simulink model "ALU_Project"  (R2023b)
settings: Solver=VariableStepAuto  StartTime=0.0  StopTime=1  RelTol=1e-3
values from neighbouring files (symbols this model uses):
  A0 = str2num(get(handles.a0i,'string'))    [AluGui.m]
  A1 = str2num(get(handles.a1i,'string'))    [AluGui.m]
  A2 = str2num(get(handles.a2i,'string'))    [AluGui.m]
  A3 = str2num(get(handles.a3i,'string'))    [AluGui.m]
  B0 = str2num(get(handles.b0i,'string'))    [AluGui.m]
  B1 = str2num(get(handles.b1i,'string'))    [AluGui.m]
  B2 = str2num(get(handles.b2i,'string'))    [AluGui.m]
  B3 = str2num(get(handles.b3i,'string'))    [AluGui.m]
  Cin = str2num(get(handles.cii,'string'))    [AluGui.m]
undefined symbols (not defined in the file or in its folder): S0, S1, S2, S3
(part 1 of 2)
settings Model: Creator=remon  LastModifiedBy=Ibrahim

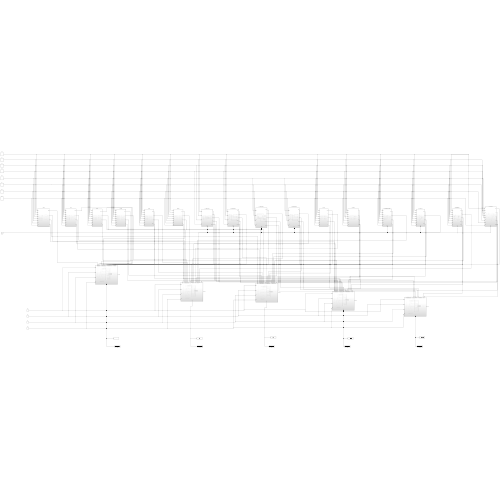
[thumbnail: Simulink's stored preview of the top-level diagram]
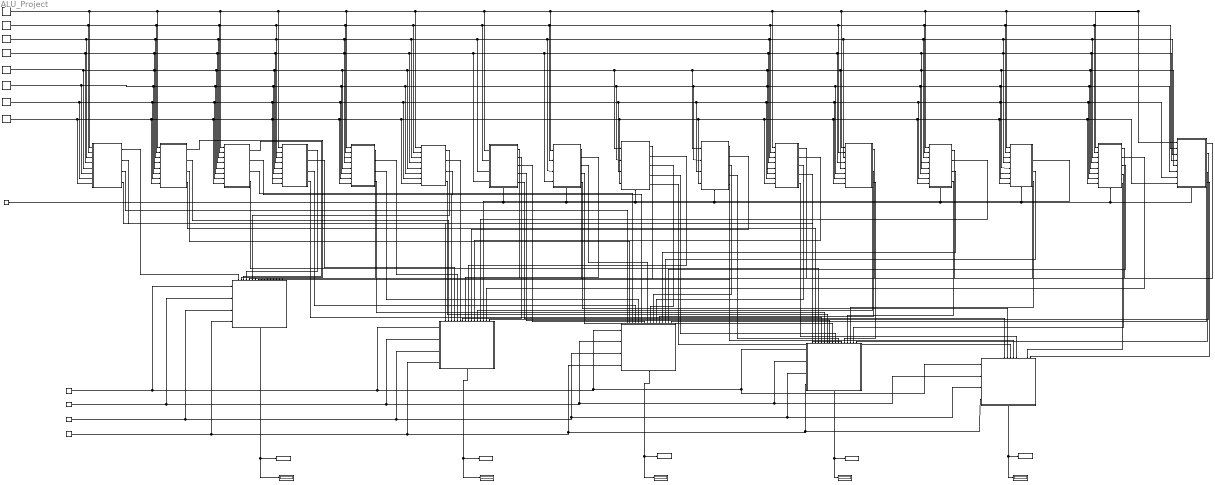
== system ALU_Project ==
  1 AND : Subsystem
  10 -SHIFT RIGHT B : Subsystem
      settings: PortSchema="{\"entries\":[{\"content\":{\"sides\":[{\"content\":{\"connectorIds\":[\"In1\",\"In2\",\"In3\",\"In4\"]},\"type\":\"ConnectorPlacement.EquallySpacedRectSide\",\"uuid\":\"67726d20-445a-49cb-8099-ac09b8ccc5e3\"},{\"content\":{\"connectorIds\":[\"Out1\",\"Out2\",\"Out3\",\"Out4\",\"Out5\"],\"side\":\"RIGHT\"},\"type\":\"ConnectorPlacement.EquallySpacedRectSide\",\"uuid\":\"ee54af08-fb8b-46dc-82ba-e86450b02724\"},{\"content\":{\"side\":\"TOP\"},\"type\":\"ConnectorPlacement.EquallySpacedRectSide\",\"uuid\":\"af06175e-2524-4fad-9974-7a0067daabff\"},{\"content\":{\"connectorIds\":[\"In5\"],\"side\":\"BOTTOM\"},\"type\":\"ConnectorPlacement.EquallySpacedRectSide\",\"uuid\":\"92107ca8-34e5-4b67-bc45-0b30bbde407d\"}]},\"type\":\"ConnectorPlacement.EquallySpacedConnector\",\"uuid\":\"fa9ce2c6-f799-4f73-a92a-f2785f87a999\"}],\"packageUris\":[\"http://schema.mathworks.com/mf0/Connector/R2020b\"],\"version\":\"1.0\"}"
  11 ADD : Subsystem
  12 Subract : Subsystem
  13- SELECTIVE CLEAR : Subsystem
      settings: PortSchema="{\"entries\":[{\"content\":{\"sides\":[{\"content\":{\"connectorIds\":[\"In1\",\"In2\",\"In3\",\"In4\",\"In5\",\"In6\",\"In7\",\"In8\"]},\"type\":\"ConnectorPlacement.EquallySpacedRectSide\",\"uuid\":\"aab1b221-1cb0-4ca9-8866-8bcfb9a4275b\"},{\"content\":{\"connectorIds\":[\"Out1\",\"Out2\",\"Out3\",\"Out4\"],\"side\":\"RIGHT\"},\"type\":\"ConnectorPlacement.EquallySpacedRectSide\",\"uuid\":\"6c2b9ce8-0a07-48e2-b787-5726e3fcf444\"},{\"content\":{\"side\":\"TOP\"},\"type\":\"ConnectorPlacement.EquallySpacedRectSide\",\"uuid\":\"ec29be9f-ac31-4973-a38d-892f27b9a585\"},{\"content\":{\"connectorIds\":[\"In9\"],\"side\":\"BOTTOM\"},\"type\":\"ConnectorPlacement.EquallySpacedRectSide\",\"uuid\":\"88a653d5-a71c-4607-949c-648803d8be5b\"}]},\"type\":\"ConnectorPlacement.EquallySpacedConnector\",\"uuid\":\"295ec8fd-c3b0-41a0-b149-0cfcf8f834a3\"}],\"packageUris\":[\"http://schema.mathworks.com/mf0/Connector/R2020b\"],\"version\":\"1.0\"}"
  14 Compleent : Subsystem
      settings: PortSchema="{\"entries\":[{\"content\":{\"sides\":[{\"content\":{\"connectorIds\":[\"In1\",\"In2\",\"In3\",\"In4\",\"In5\",\"In6\",\"In7\",\"In8\"]},\"type\":\"ConnectorPlacement.EquallySpacedRectSide\",\"uuid\":\"aab1b221-1cb0-4ca9-8866-8bcfb9a4275b\"},{\"content\":{\"connectorIds\":[\"Out1\",\"Out2\",\"Out3\",\"Out4\"],\"side\":\"RIGHT\"},\"type\":\"ConnectorPlacement.EquallySpacedRectSide\",\"uuid\":\"6c2b9ce8-0a07-48e2-b787-5726e3fcf444\"},{\"content\":{\"side\":\"TOP\"},\"type\":\"ConnectorPlacement.EquallySpacedRectSide\",\"uuid\":\"ec29be9f-ac31-4973-a38d-892f27b9a585\"},{\"content\":{\"connectorIds\":[\"In9\"],\"side\":\"BOTTOM\"},\"type\":\"ConnectorPlacement.EquallySpacedRectSide\",\"uuid\":\"df039325-7ad8-41a5-924c-b29ed495d143\"}]},\"type\":\"ConnectorPlacement.EquallySpacedConnector\",\"uuid\":\"295ec8fd-c3b0-41a0-b149-0cfcf8f834a3\"}],\"packageUris\":[\"http://schema.mathworks.com/mf0/Connector/R2020b\"],\"version\":\"1.0\"}"
  15-DECREMENT : Subsystem
      settings: PortSchema="{\"entries\":[{\"content\":{\"sides\":[{\"content\":{\"connectorIds\":[\"In1\",\"In2\",\"In3\",\"In4\",\"In5\",\"In6\",\"In7\",\"In8\"]},\"type\":\"ConnectorPlacement.EquallySpacedRectSide\",\"uuid\":\"869fb0d4-d1f3-44bd-a919-19db4d026c4c\"},{\"content\":{\"connectorIds\":[\"Out1\",\"Out2\",\"Out3\",\"Out4\",\"Out5\"],\"side\":\"RIGHT\"},\"type\":\"ConnectorPlacement.EquallySpacedRectSide\",\"uuid\":\"d1e23600-62c0-4a53-bf3f-03977fd433f6\"},{\"content\":{\"side\":\"TOP\"},\"type\":\"ConnectorPlacement.EquallySpacedRectSide\",\"uuid\":\"a43d6e83-8d01-47cf-bcfd-6ee8cba25de0\"},{\"content\":{\"connectorIds\":[\"In9\"],\"side\":\"BOTTOM\"},\"type\":\"ConnectorPlacement.EquallySpacedRectSide\",\"uuid\":\"b69fe367-260d-455e-bab1-d94656d66442\"}]},\"type\":\"ConnectorPlacement.EquallySpacedConnector\",\"uuid\":\"60700526-3682-4bd8-a800-7fae9f1c6513\"}],\"packageUris\":[\"http://schema.mathworks.com/mf0/Connector/R2020b\"],\"version\":\"1.0\"}"
  16 -Increment : Subsystem
      settings: PortSchema="{\"entries\":[{\"content\":{\"sides\":[{\"content\":{\"connectorIds\":[\"In1\",\"In2\",\"In3\",\"In4\",\"In5\",\"In6\",\"In7\",\"In8\"]},\"type\":\"ConnectorPlacement.EquallySpacedRectSide\",\"uuid\":\"3ea3efc1-2c41-45a7-8c9d-434968181f92\"},{\"content\":{\"connectorIds\":[\"Out1\",\"Out2\",\"Out3\",\"Out4\",\"Out5\"],\"side\":\"RIGHT\"},\"type\":\"ConnectorPlacement.EquallySpacedRectSide\",\"uuid\":\"65b61c40-0cda-4050-95e7-78f124d34506\"},{\"content\":{\"side\":\"TOP\"},\"type\":\"ConnectorPlacement.EquallySpacedRectSide\",\"uuid\":\"defff18e-4aec-4535-bbe1-adefcaebceb1\"},{\"content\":{\"connectorIds\":[\"In9\"],\"side\":\"BOTTOM\"},\"type\":\"ConnectorPlacement.EquallySpacedRectSide\",\"uuid\":\"2835e909-4c73-48e4-9b82-396162bc7647\"}]},\"type\":\"ConnectorPlacement.EquallySpacedConnector\",\"uuid\":\"844f857b-b7f5-4d2c-b420-0fa89070e8b7\"}],\"packageUris\":[\"http://schema.mathworks.com/mf0/Connector/R2020b\"],\"version\":\"1.0\"}"
  2 OR : Subsystem
  3 NOR : Subsystem
  4 NAND : Subsystem
  5 XOR : Subsystem
  6 XNOR : Subsystem
  7 - A SHFIT LEFT : Subsystem
      settings: PortSchema="{\"entries\":[{\"content\":{\"sides\":[{\"content\":{\"connectorIds\":[\"In1\",\"In2\",\"In3\",\"In4\"]},\"type\":\"ConnectorPlacement.EquallySpacedRectSide\",\"uuid\":\"67726d20-445a-49cb-8099-ac09b8ccc5e3\"},{\"content\":{\"connectorIds\":[\"Out1\",\"Out2\",\"Out3\",\"Out4\",\"Out5\"],\"side\":\"RIGHT\"},\"type\":\"ConnectorPlacement.EquallySpacedRectSide\",\"uuid\":\"ee54af08-fb8b-46dc-82ba-e86450b02724\"},{\"content\":{\"side\":\"TOP\"},\"type\":\"ConnectorPlacement.EquallySpacedRectSide\",\"uuid\":\"af06175e-2524-4fad-9974-7a0067daabff\"},{\"content\":{\"connectorIds\":[\"In5\"],\"side\":\"BOTTOM\"},\"type\":\"ConnectorPlacement.EquallySpacedRectSide\",\"uuid\":\"f9a8dd3b-7a22-45bd-9502-add1c2d213e4\"}]},\"type\":\"ConnectorPlacement.EquallySpacedConnector\",\"uuid\":\"fa9ce2c6-f799-4f73-a92a-f2785f87a999\"}],\"packageUris\":[\"http://schema.mathworks.com/mf0/Connector/R2020b\"],\"version\":\"1.0\"}"
  8 - SHIFT RIGHT A : Subsystem
      settings: PortSchema="{\"entries\":[{\"content\":{\"sides\":[{\"content\":{\"connectorIds\":[\"In1\",\"In2\",\"In3\",\"In4\"]},\"type\":\"ConnectorPlacement.EquallySpacedRectSide\",\"uuid\":\"67726d20-445a-49cb-8099-ac09b8ccc5e3\"},{\"content\":{\"connectorIds\":[\"Out1\",\"Out2\",\"Out3\",\"Out4\",\"Out5\"],\"side\":\"RIGHT\"},\"type\":\"ConnectorPlacement.EquallySpacedRectSide\",\"uuid\":\"ee54af08-fb8b-46dc-82ba-e86450b02724\"},{\"content\":{\"side\":\"TOP\"},\"type\":\"ConnectorPlacement.EquallySpacedRectSide\",\"uuid\":\"af06175e-2524-4fad-9974-7a0067daabff\"},{\"content\":{\"connectorIds\":[\"In5\"],\"side\":\"BOTTOM\"},\"type\":\"ConnectorPlacement.EquallySpacedRectSide\",\"uuid\":\"c41446c6-b653-4be8-be63-43ab09cffb18\"}]},\"type\":\"ConnectorPlacement.EquallySpacedConnector\",\"uuid\":\"fa9ce2c6-f799-4f73-a92a-f2785f87a999\"}],\"packageUris\":[\"http://schema.mathworks.com/mf0/Connector/R2020b\"],\"version\":\"1.0\"}"
  "9 - B SHIFT LEFT " : Subsystem
      settings: PortSchema="{\"entries\":[{\"content\":{\"sides\":[{\"content\":{\"connectorIds\":[\"In1\",\"In2\",\"In3\",\"In4\"]},\"type\":\"ConnectorPlacement.EquallySpacedRectSide\",\"uuid\":\"67726d20-445a-49cb-8099-ac09b8ccc5e3\"},{\"content\":{\"connectorIds\":[\"Out1\",\"Out2\",\"Out3\",\"Out4\",\"Out5\"],\"side\":\"RIGHT\"},\"type\":\"ConnectorPlacement.EquallySpacedRectSide\",\"uuid\":\"ee54af08-fb8b-46dc-82ba-e86450b02724\"},{\"content\":{\"side\":\"TOP\"},\"type\":\"ConnectorPlacement.EquallySpacedRectSide\",\"uuid\":\"af06175e-2524-4fad-9974-7a0067daabff\"},{\"content\":{\"connectorIds\":[\"In5\"],\"side\":\"BOTTOM\"},\"type\":\"ConnectorPlacement.EquallySpacedRectSide\",\"uuid\":\"689fe6fd-fd8e-4c12-8b2b-d8e14b2aa840\"}]},\"type\":\"ConnectorPlacement.EquallySpacedConnector\",\"uuid\":\"fa9ce2c6-f799-4f73-a92a-f2785f87a999\"}],\"packageUris\":[\"http://schema.mathworks.com/mf0/Connector/R2020b\"],\"version\":\"1.0\"}"
  A0 : Constant  Value=A0
  A1 : Constant  Value=A1
  A2 : Constant  Value=A2
  A3 : Constant  Value=A3
  B0 : Constant  Value=B0
  B1 : Constant  Value=B1
  B2 : Constant  Value=B2
  B3 : Constant  Value=B3
  CIn : Constant  Value=Cin
  Cout : Display
  S0 : Constant  Value=S0
  S1 : Constant  Value=S1
  S2 : Constant  Value=S2
  S3 : Constant  Value=S3
  To Workspace : ToWorkspace  VariableName=Z2  SampleTime=-1
  To Workspace1 : ToWorkspace  VariableName=Z3  SampleTime=-1
  To Workspace2 : ToWorkspace  VariableName=Cout  SampleTime=-1
  To Workspace3 : ToWorkspace  VariableName=Z1  SampleTime=-1
  To Workspace4 : ToWorkspace  VariableName=Z0  SampleTime=-1
  Z0 : Display
  "Z1 " : Display
  Z2 : Display
  Z3 : Display
  bit 1 out : Subsystem
      settings: PortSchema="{\"entries\":[{\"content\":{\"sides\":[{\"content\":{\"connectorIds\":[\"In1\",\"In2\",\"In3\",\"In4\",\"In5\",\"In6\",\"In7\",\"In8\",\"In9\",\"In10\",\"In11\",\"In12\",\"In13\",\"In14\",\"In15\",\"In16\"]},\"type\":\"ConnectorPlacement.EquallySpacedRectSide\",\"uuid\":\"53e370e5-cc10-417f-a084-3353bc2b3524\"},{\"content\":{\"connectorIds\":[\"Out1\"],\"side\":\"RIGHT\"},\"type\":\"ConnectorPlacement.EquallySpacedRectSide\",\"uuid\":\"f2d13301-e5be-4569-a8f2-18325db28854\"},{\"content\":{\"connectorIds\":[\"In17\",\"In18\",\"In19\",\"In20\"],\"side\":\"TOP\"},\"type\":\"ConnectorPlacement.EquallySpacedRectSide\",\"uuid\":\"c3b20576-f5d0-4622-8370-994c765f463a\"}]},\"type\":\"ConnectorPlacement.EquallySpacedConnector\",\"uuid\":\"4e1c3be4-ed9a-414f-b6f4-4528b145bb15\"}],\"packageUris\":[\"http://schema.mathworks.com/mf0/Connector/R2020b\"],\"version\":\"1.0\"}"
  bit 2 out : Subsystem
      settings: PortSchema="{\"entries\":[{\"content\":{\"sides\":[{\"content\":{\"connectorIds\":[\"In1\",\"In2\",\"In3\",\"In4\",\"In5\",\"In6\",\"In7\",\"In8\",\"In9\",\"In10\",\"In11\",\"In12\",\"In13\",\"In14\",\"In15\",\"In16\"]},\"type\":\"ConnectorPlacement.EquallySpacedRectSide\",\"uuid\":\"53e370e5-cc10-417f-a084-3353bc2b3524\"},{\"content\":{\"connectorIds\":[\"Out1\"],\"side\":\"RIGHT\"},\"type\":\"ConnectorPlacement.EquallySpacedRectSide\",\"uuid\":\"f2d13301-e5be-4569-a8f2-18325db28854\"},{\"content\":{\"connectorIds\":[\"In17\",\"In18\",\"In19\",\"In20\"],\"side\":\"TOP\"},\"type\":\"ConnectorPlacement.EquallySpacedRectSide\",\"uuid\":\"c3b20576-f5d0-4622-8370-994c765f463a\"}]},\"type\":\"ConnectorPlacement.EquallySpacedConnector\",\"uuid\":\"4e1c3be4-ed9a-414f-b6f4-4528b145bb15\"}],\"packageUris\":[\"http://schema.mathworks.com/mf0/Connector/R2020b\"],\"version\":\"1.0\"}"
  bit 3 out : Subsystem
      settings: PortSchema="{\"entries\":[{\"content\":{\"sides\":[{\"content\":{\"connectorIds\":[\"In1\",\"In2\",\"In3\",\"In4\",\"In5\",\"In6\",\"In7\",\"In8\",\"In9\",\"In10\",\"In11\",\"In12\",\"In13\",\"In14\",\"In15\",\"In16\"]},\"type\":\"ConnectorPlacement.EquallySpacedRectSide\",\"uuid\":\"53e370e5-cc10-417f-a084-3353bc2b3524\"},{\"content\":{\"connectorIds\":[\"Out1\"],\"side\":\"RIGHT\"},\"type\":\"ConnectorPlacement.EquallySpacedRectSide\",\"uuid\":\"f2d13301-e5be-4569-a8f2-18325db28854\"},{\"content\":{\"connectorIds\":[\"In17\",\"In18\",\"In19\",\"In20\"],\"side\":\"TOP\"},\"type\":\"ConnectorPlacement.EquallySpacedRectSide\",\"uuid\":\"c3b20576-f5d0-4622-8370-994c765f463a\"}]},\"type\":\"ConnectorPlacement.EquallySpacedConnector\",\"uuid\":\"4e1c3be4-ed9a-414f-b6f4-4528b145bb15\"}],\"packageUris\":[\"http://schema.mathworks.com/mf0/Connector/R2020b\"],\"version\":\"1.0\"}"
  bit 4 out : Subsystem
      settings: PortSchema="{\"entries\":[{\"content\":{\"sides\":[{\"content\":{\"connectorIds\":[\"In1\",\"In2\",\"In3\",\"In4\",\"In5\",\"In6\",\"In7\",\"In8\",\"In9\",\"In10\",\"In11\",\"In12\",\"In13\",\"In14\",\"In15\",\"In16\"]},\"type\":\"ConnectorPlacement.EquallySpacedRectSide\",\"uuid\":\"53e370e5-cc10-417f-a084-3353bc2b3524\"},{\"content\":{\"connectorIds\":[\"Out1\"],\"side\":\"RIGHT\"},\"type\":\"ConnectorPlacement.EquallySpacedRectSide\",\"uuid\":\"f2d13301-e5be-4569-a8f2-18325db28854\"},{\"content\":{\"connectorIds\":[\"In17\",\"In18\",\"In19\",\"In20\"],\"side\":\"TOP\"},\"type\":\"ConnectorPlacement.EquallySpacedRectSide\",\"uuid\":\"c3b20576-f5d0-4622-8370-994c765f463a\"}]},\"type\":\"ConnectorPlacement.EquallySpacedConnector\",\"uuid\":\"4e1c3be4-ed9a-414f-b6f4-4528b145bb15\"}],\"packageUris\":[\"http://schema.mathworks.com/mf0/Connector/R2020b\"],\"version\":\"1.0\"}"
  bit Cout : Subsystem
      settings: PortSchema="{\"entries\":[{\"content\":{\"sides\":[{\"content\":{\"connectorIds\":[\"In1\",\"In2\",\"In3\",\"In4\",\"In5\",\"In6\",\"In7\",\"In8\",\"In9\",\"In10\",\"In11\",\"In12\",\"In13\",\"In14\",\"In15\",\"In16\"]},\"type\":\"ConnectorPlacement.EquallySpacedRectSide\",\"uuid\":\"53e370e5-cc10-417f-a084-3353bc2b3524\"},{\"content\":{\"connectorIds\":[\"Out1\"],\"side\":\"RIGHT\"},\"type\":\"ConnectorPlacement.EquallySpacedRectSide\",\"uuid\":\"f2d13301-e5be-4569-a8f2-18325db28854\"},{\"content\":{\"connectorIds\":[\"In17\",\"In18\",\"In19\",\"In20\"],\"side\":\"TOP\"},\"type\":\"ConnectorPlacement.EquallySpacedRectSide\",\"uuid\":\"c3b20576-f5d0-4622-8370-994c765f463a\"}]},\"type\":\"ConnectorPlacement.EquallySpacedConnector\",\"uuid\":\"4e1c3be4-ed9a-414f-b6f4-4528b145bb15\"}],\"packageUris\":[\"http://schema.mathworks.com/mf0/Connector/R2020b\"],\"version\":\"1.0\"}"
  wires:
  B1/1 -> 1 AND/6(B1), 2 OR/6(B1), 4 NAND/6(B1), 5 XOR/6(B1), 6 XNOR/6(B1), "9 - B SHIFT LEFT "/2(B1), 10 -SHIFT RIGHT B/2(B1), 11 ADD/6(B1), 12 Subract/6(B1), 13- SELECTIVE CLEAR/6(B1), 14 Compleent/6(B1), 15-DECREMENT/6(B1), 16 -Increment/6(B1), 3 NOR/6(B1)
  A3/1 -> 1 AND/4(A3), 2 OR/4(A3), 4 NAND/4(A3), 5 XOR/4(A3), 6 XNOR/4(A3), 7 - A SHFIT LEFT/4(A3), 8 - SHIFT RIGHT A/4(A3), 11 ADD/4(A3), 12 Subract/4(A3), 13- SELECTIVE CLEAR/4(A3), 14 Compleent/4(A3), 15-DECREMENT/4(A3), 16 -Increment/4(A3), 3 NOR/4(A3)
  B3/1 -> 1 AND/8(B3), 2 OR/8(B3), 4 NAND/8(B3), 6 XNOR/8(B3), "9 - B SHIFT LEFT "/4(B3), 10 -SHIFT RIGHT B/4(B3), 11 ADD/8(B3), 12 Subract/8(B3), 13- SELECTIVE CLEAR/8(B3), 14 Compleent/8(B3), 15-DECREMENT/8(B3), 16 -Increment/8(B3), 5 XOR/8(B3), 3 NOR/8(B3)
  B2/1 -> 1 AND/7(B2), 2 OR/7(B2), 4 NAND/7(B2), 5 XOR/7(B2), 6 XNOR/7(B2), "9 - B SHIFT LEFT "/3(B2), 10 -SHIFT RIGHT B/3(B2), 11 ADD/7(B2), 12 Subract/7(B2), 13- SELECTIVE CLEAR/7(B2), 14 Compleent/7(B2), 15-DECREMENT/7(B2), 16 -Increment/7(B2), 3 NOR/7(B2)
  A1/1 -> 1 AND/2(A1), 2 OR/2(A1), 4 NAND/2(A1), 6 XNOR/2(A1), 7 - A SHFIT LEFT/2(A1), 8 - SHIFT RIGHT A/2(A1), 13- SELECTIVE CLEAR/2(A1), 16 -Increment/2(A1), 15-DECREMENT/2(A1), 14 Compleent/2(A1), 12 Subract/2(A1), 11 ADD/2(A1), 5 XOR/2(A1), 3 NOR/2(A1)
  B0/1 -> 1 AND/5(B0), 2 OR/5(B0), 4 NAND/5(B0), 5 XOR/5(B0), 6 XNOR/5(B0), "9 - B SHIFT LEFT "/1(B0), 10 -SHIFT RIGHT B/1(B0), 11 ADD/5(B0), 14 Compleent/5(B0), 15-DECREMENT/5(B0), 16 -Increment/5(B0), 13- SELECTIVE CLEAR/5(B0), 12 Subract/5(B0), 3 NOR/5(B0)
  A2/1 -> 1 AND/3(A2), 2 OR/3(A2), 4 NAND/3(A2), 5 XOR/3(A2), 6 XNOR/3(A2), 7 - A SHFIT LEFT/3(A2), 8 - SHIFT RIGHT A/3(A2), 11 ADD/3(A2), 12 Subract/3(A2), 14 Compleent/3(A2), 15-DECREMENT/3(A2), 16 -Increment/3(A2), 13- SELECTIVE CLEAR/3(A2), 3 NOR/3(A2)
  A0/1 -> 1 AND/1(A0), 2 OR/1(A0), 4 NAND/1(A0), 5 XOR/1(A0), 6 XNOR/1(A0), 7 - A SHFIT LEFT/1(A0), 8 - SHIFT RIGHT A/1(A0), 11 ADD/1(A0), 12 Subract/1(A0), 13- SELECTIVE CLEAR/1(A0), 14 Compleent/1(A0), 16 -Increment/1(A0), 15-DECREMENT/1(A0), 3 NOR/1(A0)
  CIn/1 -> 8 - SHIFT RIGHT A/5(CIN), 13- SELECTIVE CLEAR/9(CIN), 16 -Increment/9(Cin), 15-DECREMENT/9(Cin), 14 Compleent/9(Cin), 10 -SHIFT RIGHT B/5(CIN), "9 - B SHIFT LEFT "/5(CIN), 7 - A SHFIT LEFT/5(CIN)
  1 AND/1(0000) -> bit 1 out/1(0000)
  2 OR/1(0001) -> bit 1 out/2(0001)
  3 NOR/1(0010) -> bit 1 out/3(0010)
  4 NAND/1(0011) -> bit 1 out/4(0011)
  5 XOR/1(0100) -> bit 1 out/5(0100)
  6 XNOR/1(0101) -> bit 1 out/6(0101)
  7 - A SHFIT LEFT/1(1) -> bit 1 out/7(0110)
  8 - SHIFT RIGHT A/1(0111) -> bit 1 out/8(0111)
  "9 - B SHIFT LEFT "/1(1000) -> bit 1 out/9(1000)
  10 -SHIFT RIGHT B/1(1001) -> bit 1 out/10(1001)
  11 ADD/1(1010) -> bit 1 out/11(1010)
  12 Subract/1(1) -> bit 1 out/12(1011)
  13- SELECTIVE CLEAR/1(1100) -> bit 1 out/13(1100)
  14 Compleent/1(1101) -> bit 1 out/14(1101)
  15-DECREMENT/1(1110) -> bit 1 out/15(1110)
  16 -Increment/1(1111) -> bit 1 out/16(1111)
  1 AND/2(Out2) -> bit 2 out/1(0000)
  2 OR/2(Out2) -> bit 2 out/2(0001)
  3 NOR/2(Out2) -> bit 2 out/3(0010)
  4 NAND/2(Out2) -> bit 2 out/4(0011)
  5 XOR/2(Out2) -> bit 2 out/5(0100)
  6 XNOR/2(Out2) -> bit 2 out/6(0101)
  7 - A SHFIT LEFT/2(2) -> bit 2 out/7(0110)
  8 - SHIFT RIGHT A/2(Out2) -> bit 2 out/8(0111)
  "9 - B SHIFT LEFT "/2(Out2) -> bit 2 out/9(1000)
  10 -SHIFT RIGHT B/2(Out2) -> bit 2 out/10(1001)
  11 ADD/2(Out2) -> bit 2 out/11(1010)
  12 Subract/2(Out2) -> bit 2 out/12(1011)
  13- SELECTIVE CLEAR/2(Out2) -> bit 2 out/13(1100)
  14 Compleent/2(Out2) -> bit 2 out/14(1101)
  15-DECREMENT/2(Out2) -> bit 2 out/15(1110)
  16 -Increment/2(Out2) -> bit 2 out/16(1111)
  1 AND/3(Out3) -> bit 3 out/1(0000)
  2 OR/3(Out3) -> bit 3 out/2(0001)
  3 NOR/3(Out3) -> bit 3 out/3(0010)
  4 NAND/3(Out3) -> bit 3 out/4(0011)
  5 XOR/3(Out3) -> bit 3 out/5(0100)
  6 XNOR/3(Out3) -> bit 3 out/6(0101)
  7 - A SHFIT LEFT/3(3) -> bit 3 out/7(0110)
  8 - SHIFT RIGHT A/3(Out3) -> bit 3 out/8(0111)
  "9 - B SHIFT LEFT "/3(Out3) -> bit 3 out/9(1000)
  10 -SHIFT RIGHT B/3(Out3) -> bit 3 out/10(1001)
  11 ADD/3(Out3) -> bit 3 out/11(1010)
  12 Subract/3(Out3) -> bit 3 out/12(1011)
  13- SELECTIVE CLEAR/3(Out3) -> bit 3 out/13(1100)
  14 Compleent/3(Out3) -> bit 3 out/14(1101)
  15-DECREMENT/3(Out3) -> bit 3 out/15(1110)
  16 -Increment/3(Out3) -> bit 3 out/16(1111)
  1 AND/4(Out4) -> bit 4 out/1(0000)
  2 OR/4(Out4) -> bit 4 out/2(0001)
  3 NOR/4(Out4) -> bit 4 out/3(0010)
  4 NAND/4(Out4) -> bit 4 out/4(0011)
  5 XOR/4(0101) -> bit 4 out/5(0100)
  6 XNOR/4(Out4) -> bit 4 out/6(0101)
  7 - A SHFIT LEFT/4(" 4") -> bit 4 out/7(0110)
  8 - SHIFT RIGHT A/4(Out 4) -> bit 4 out/8(0111)
  "9 - B SHIFT LEFT "/4(Out 4) -> bit 4 out/9(1000)
  10 -SHIFT RIGHT B/4(Out 4) -> bit 4 out/10(1001)
  11 ADD/4(Out4) -> bit 4 out/11(1010)
  12 Subract/4(Out4) -> bit 4 out/12(1011)
  13- SELECTIVE CLEAR/4(Out4) -> bit 4 out/13(1100)
  14 Compleent/4(1100) -> bit 4 out/14(1101)
  15-DECREMENT/4(1101) -> bit 4 out/15(1110)
  16 -Increment/4(Out4) -> bit 4 out/16(1111)
  7 - A SHFIT LEFT/5(COUT) -> bit Cout/7(0110)
  8 - SHIFT RIGHT A/5(COUT) -> bit Cout/8(0111)
  "9 - B SHIFT LEFT "/5(COUT) -> bit Cout/9(1000)
  10 -SHIFT RIGHT B/5(COUT) -> bit Cout/10(1001)
  15-DECREMENT/5(Cout) -> bit Cout/15(1110)
  16 -Increment/5(Cout) -> bit Cout/16(1111)
  bit Cout/1(Out) -> Cout/1, To Workspace2/1
  bit 4 out/1(Out) -> To Workspace1/1, Z3/1
  bit 3 out/1(Out) -> To Workspace/1, Z2/1
  bit 2 out/1(Out) -> To Workspace3/1, "Z1 "/1
  bit 1 out/1(Out) -> To Workspace4/1, Z0/1
  S3/1 -> bit 1 out/17(S3), bit 2 out/17(S3), bit Cout/17(S3), bit 4 out/17(S3), bit 3 out/17(S3)
  S2/1 -> bit 1 out/18(S2), bit 2 out/18(S2), bit Cout/18(S2), bit 4 out/18(S2), bit 3 out/18(S2)
  S1/1 -> bit 1 out/19(S1), bit 2 out/19(S1), bit 3 out/19(S1), bit Cout/19(S1), bit 4 out/19(S1)
  S0/1 -> bit 2 out/20(S0), bit 3 out/20(S0), bit 4 out/20(S0), bit Cout/20(S0), bit 1 out/20(S0)
  11 ADD/5(Out5) -> bit Cout/11(1010)

== system ALU_Project/1 AND ==
  A0 : Inport
  A1 : Inport  Port=2
  A2 : Inport  Port=3
  A3 : Inport  Port=4
  B0 : Inport  Port=5
  B1 : Inport  Port=6
  B2 : Inport  Port=7
  B3 : Inport  Port=8
   {,1..3} (4 alike) : Logic  AllPortsSameDT=off  OutDataTypeStr=boolean
  display{,1..3} (4 alike) : Display
  0000 : Outport
  Out2 : Outport  Port=2
  Out3 : Outport  Port=3
  Out4 : Outport  Port=4
  wires:
  A0/1 -> " "/1
  B0/1 -> " "/2
  A1/1 -> " 1"/1
  B1/1 -> " 1"/2
  A2/1 -> " 2"/1
  B2/1 -> " 2"/2
  A3/1 -> " 3"/1
  B3/1 -> " 3"/2
  " 1"/1 -> Out2/1, display1/1
  " "/1 -> 0000/1, display/1
  " 3"/1 -> Out4/1, display3/1
  " 2"/1 -> Out3/1, display2/1

== system ALU_Project/10 -SHIFT RIGHT B ==
  B0 : Inport
  B1 : Inport  Port=2
  B2 : Inport  Port=3
  B3 : Inport  Port=4
  CIN : Inport  Port=5
  1001 : Outport
  Out2 : Outport  Port=2
  Out3 : Outport  Port=3
  Out 4 : Outport  Port=4
  COUT : Outport  Port=5
  wires:
  B3/1 -> Out3/1
  CIN/1 -> Out 4/1
  B2/1 -> Out2/1
  B1/1 -> 1001/1
  B0/1 -> COUT/1

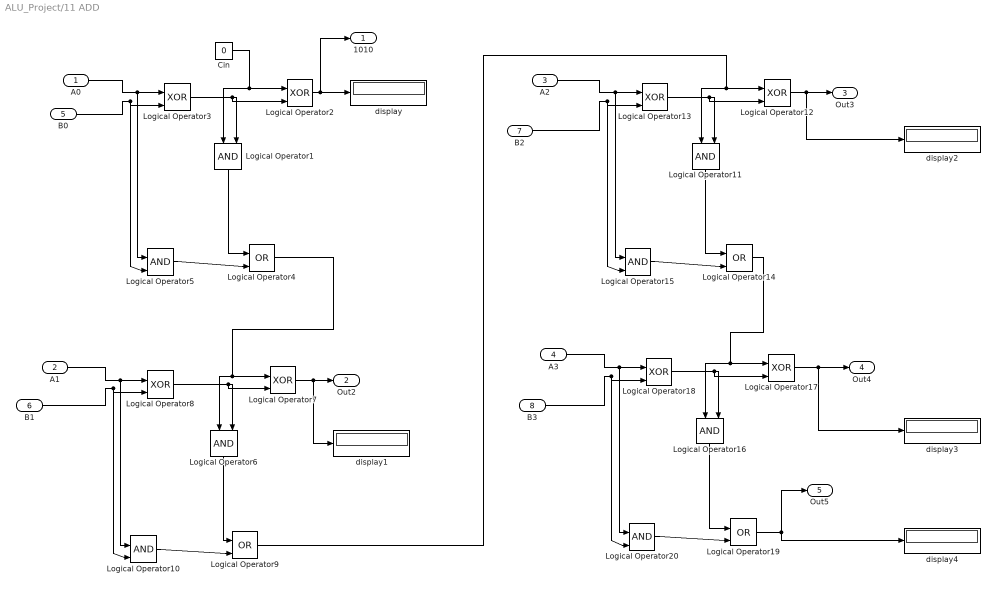
== system ALU_Project/11 ADD ==
  A0 : Inport
  A1 : Inport  Port=2
  A2 : Inport  Port=3
  A3 : Inport  Port=4
  B0 : Inport  Port=5
  B1 : Inport  Port=6
  B2 : Inport  Port=7
  B3 : Inport  Port=8
  Cin : Constant  Value=0
  Logical Operator{1,5..6,10..11,15..16,20} (8 alike) : Logic  IconShape=distinctive  AllPortsSameDT=off  OutDataTypeStr=boolean
  Logical Operator{2..3,7..8,12..13,17..18} (8 alike) : Logic  Operator=XOR  IconShape=distinctive  AllPortsSameDT=off  OutDataTypeStr=boolean
  Logical Operator{4,9,14,19} (4 alike) : Logic  Operator=OR  IconShape=distinctive  AllPortsSameDT=off  OutDataTypeStr=boolean
  display{,1..4} (5 alike) : Display
  1010 : Outport
  Out2 : Outport  Port=2
  Out3 : Outport  Port=3
  Out4 : Outport  Port=4
  Out5 : Outport  Port=5
  wires:
  Logical Operator3/1 -> Logical Operator2/2, Logical Operator1/2
  Logical Operator1/1 -> Logical Operator4/1
  Logical Operator5/1 -> Logical Operator4/2
  B0/1 -> Logical Operator5/2, Logical Operator3/2
  Cin/1 -> Logical Operator1/1, Logical Operator2/1
  Logical Operator2/1 -> display/1, 1010/1
  A0/1 -> Logical Operator5/1, Logical Operator3/1
  Logical Operator8/1 -> Logical Operator7/2, Logical Operator6/2
  Logical Operator6/1 -> Logical Operator9/1
  Logical Operator10/1 -> Logical Operator9/2
  B1/1 -> Logical Operator10/2, Logical Operator8/2
  Logical Operator4/1 -> Logical Operator6/1, Logical Operator7/1
  Logical Operator7/1 -> display1/1, Out2/1
  A1/1 -> Logical Operator10/1, Logical Operator8/1
  Logical Operator13/1 -> Logical Operator12/2, Logical Operator11/2
  Logical Operator11/1 -> Logical Operator14/1
  Logical Operator15/1 -> Logical Operator14/2
  B2/1 -> Logical Operator15/2, Logical Operator13/2
  Logical Operator9/1 -> Logical Operator11/1, Logical Operator12/1
  A2/1 -> Logical Operator15/1, Logical Operator13/1
  Logical Operator18/1 -> Logical Operator17/2, Logical Operator16/2
  Logical Operator16/1 -> Logical Operator19/1
  Logical Operator20/1 -> Logical Operator19/2
  B3/1 -> Logical Operator20/2, Logical Operator18/2
  Logical Operator14/1 -> Logical Operator16/1, Logical Operator17/1
  A3/1 -> Logical Operator20/1, Logical Operator18/1
  Logical Operator12/1 -> display2/1, Out3/1
  Logical Operator17/1 -> display3/1, Out4/1
  Logical Operator19/1 -> Out5/1, display4/1

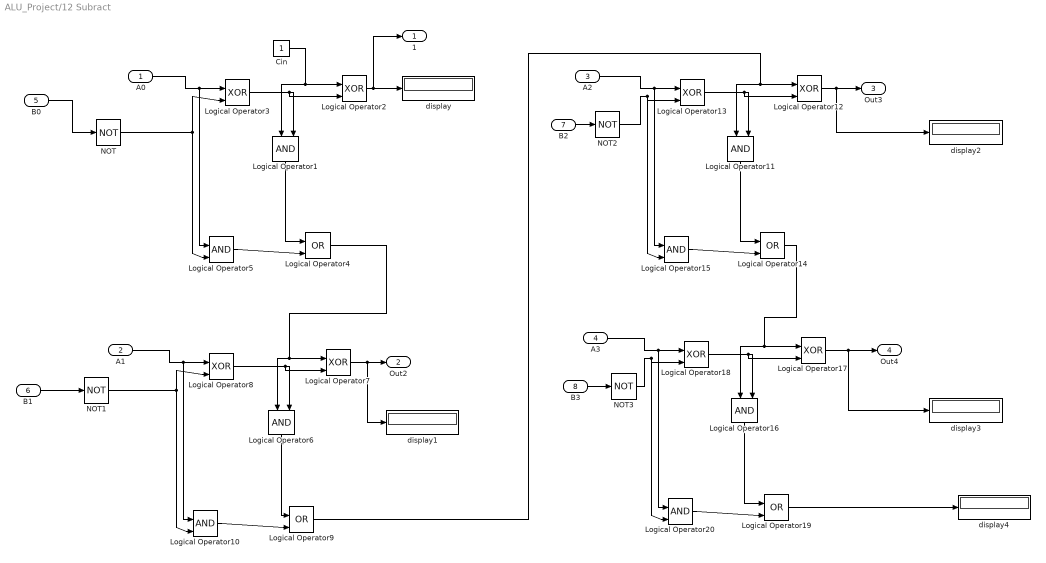
== system ALU_Project/12 Subract ==
  A0 : Inport
  A1 : Inport  Port=2
  A2 : Inport  Port=3
  A3 : Inport  Port=4
  B0 : Inport  Port=5
  B1 : Inport  Port=6
  B2 : Inport  Port=7
  B3 : Inport  Port=8
  Cin : Constant
  Logical Operator{1,5..6,10..11,15..16,20} (8 alike) : Logic  IconShape=distinctive  AllPortsSameDT=off  OutDataTypeStr=boolean
  Logical Operator{2..3,7..8,12..13,17..18} (8 alike) : Logic  Operator=XOR  IconShape=distinctive  AllPortsSameDT=off  OutDataTypeStr=boolean
  Logical Operator{4,9,14,19} (4 alike) : Logic  Operator=OR  IconShape=distinctive  AllPortsSameDT=off  OutDataTypeStr=boolean
  NOT{,1..3} (4 alike) : Logic  Operator=NOT  IconShape=distinctive  AllPortsSameDT=off  OutDataTypeStr=boolean
  display{,1..4} (5 alike) : Display
  1 : Outport
  Out2 : Outport  Port=2
  Out3 : Outport  Port=3
  Out4 : Outport  Port=4
  wires:
  Logical Operator9/1 -> Logical Operator11/1, Logical Operator12/1
  A3/1 -> Logical Operator20/1, Logical Operator18/1
  Logical Operator7/1 -> display1/1, Out2/1
  A0/1 -> Logical Operator5/1, Logical Operator3/1
  B2/1 -> NOT2/1
  Logical Operator14/1 -> Logical Operator16/1, Logical Operator17/1
  B3/1 -> NOT3/1
  A1/1 -> Logical Operator10/1, Logical Operator8/1
  Logical Operator19/1 -> display4/1
  Logical Operator4/1 -> Logical Operator6/1, Logical Operator7/1
  Logical Operator12/1 -> display2/1, Out3/1
  Logical Operator13/1 -> Logical Operator12/2, Logical Operator11/2
  Logical Operator16/1 -> Logical Operator19/1
  Logical Operator18/1 -> Logical Operator17/2, Logical Operator16/2
  A2/1 -> Logical Operator15/1, Logical Operator13/1
  Logical Operator8/1 -> Logical Operator7/2, Logical Operator6/2
  B1/1 -> NOT1/1
  Logical Operator15/1 -> Logical Operator14/2
  Logical Operator11/1 -> Logical Operator14/1
  Logical Operator5/1 -> Logical Operator4/2
  Logical Operator3/1 -> Logical Operator2/2, Logical Operator1/2
  Cin/1 -> Logical Operator1/1, Logical Operator2/1
  Logical Operator10/1 -> Logical Operator9/2
  Logical Operator17/1 -> display3/1, Out4/1
  Logical Operator20/1 -> Logical Operator19/2
  Logical Operator6/1 -> Logical Operator9/1
  B0/1 -> NOT/1
  Logical Operator1/1 -> Logical Operator4/1
  Logical Operator2/1 -> display/1, 1/1
  NOT/1 -> Logical Operator3/2, Logical Operator5/2
  NOT1/1 -> Logical Operator8/2, Logical Operator10/2
  NOT2/1 -> Logical Operator15/2, Logical Operator13/2
  NOT3/1 -> Logical Operator20/2, Logical Operator18/2

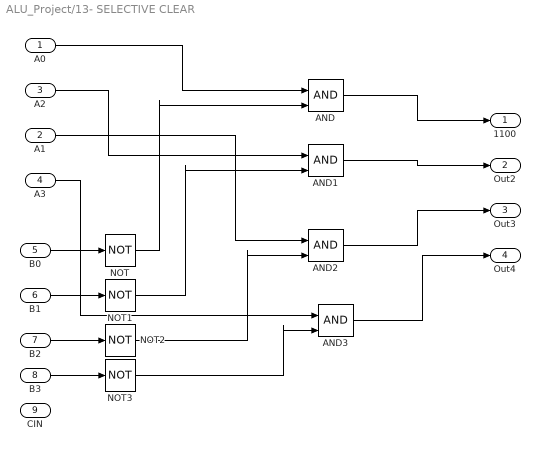
== system ALU_Project/13- SELECTIVE CLEAR ==
  A0 : Inport
  A1 : Inport  Port=2
  A2 : Inport  Port=3
  A3 : Inport  Port=4
  B0 : Inport  Port=5
  B1 : Inport  Port=6
  B2 : Inport  Port=7
  B3 : Inport  Port=8
  CIN : Inport  Port=9
  AND{,1..3} (4 alike) : Logic  IconShape=distinctive  AllPortsSameDT=off  OutDataTypeStr=boolean
  NOT{,1..3} (4 alike) : Logic  Operator=NOT  IconShape=distinctive  AllPortsSameDT=off  OutDataTypeStr=boolean
  1100 : Outport
  Out2 : Outport  Port=2
  Out3 : Outport  Port=3
  Out4 : Outport  Port=4
  wires:
  B0/1 -> NOT/1
  B1/1 -> NOT1/1
  B2/1 -> NOT2/1
  A0/1 -> AND/1
  NOT/1 -> AND/2
  A2/1 -> AND1/1
  NOT1/1 -> AND1/2
  A1/1 -> AND2/1
  A3/1 -> AND3/1
  NOT2/1 -> AND2/2
  NOT3/1 -> AND3/2
  B3/1 -> NOT3/1
  AND1/1 -> Out2/1
  AND/1 -> 1100/1
  AND2/1 -> Out3/1
  AND3/1 -> Out4/1

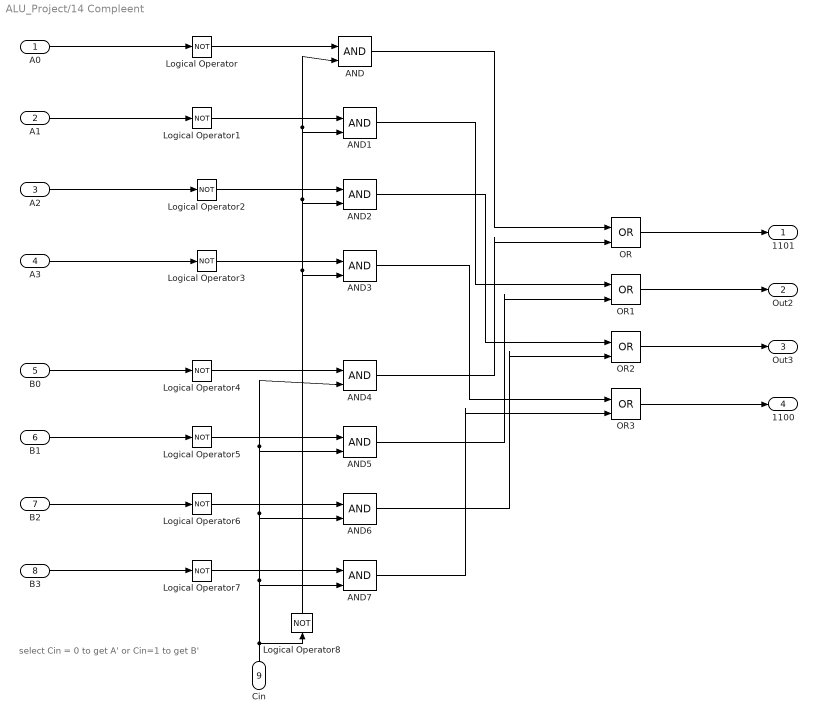
== system ALU_Project/14 Compleent ==
  note: select Cin = 0 to get A' or Cin=1 to get B'
  A0 : Inport
  A1 : Inport  Port=2
  A2 : Inport  Port=3
  A3 : Inport  Port=4
  B0 : Inport  Port=5
  B1 : Inport  Port=6
  B2 : Inport  Port=7
  B3 : Inport  Port=8
  Cin : Inport  Port=9
  AND{,1..7} (8 alike) : Logic  IconShape=distinctive  AllPortsSameDT=off  OutDataTypeStr=boolean
  Logical Operator{,1..8} (9 alike) : Logic  Operator=NOT  IconShape=distinctive  AllPortsSameDT=off  OutDataTypeStr=boolean
  OR{,1..3} (4 alike) : Logic  Operator=OR  IconShape=distinctive  AllPortsSameDT=off  OutDataTypeStr=boolean
  1101 : Outport
  Out2 : Outport  Port=2
  Out3 : Outport  Port=3
  1100 : Outport  Port=4
  wires:
  A0/1 -> Logical Operator/1
  A1/1 -> Logical Operator1/1
  A2/1 -> Logical Operator2/1
  A3/1 -> Logical Operator3/1
  B0/1 -> Logical Operator4/1
  B1/1 -> Logical Operator5/1
  B2/1 -> Logical Operator6/1
  B3/1 -> Logical Operator7/1
  Logical Operator/1 -> AND/1
  Logical Operator1/1 -> AND1/1
  Logical Operator2/1 -> AND2/1
  Logical Operator3/1 -> AND3/1
  Logical Operator4/1 -> AND4/1
  Logical Operator5/1 -> AND5/1
  Logical Operator6/1 -> AND6/1
  Logical Operator7/1 -> AND7/1
  Logical Operator8/1 -> AND3/2, AND2/2, AND1/2, AND/2
  Cin/1 -> Logical Operator8/1, AND7/2, AND6/2, AND4/2, AND5/2
  OR/1 -> 1101/1
  OR1/1 -> Out2/1
  OR2/1 -> Out3/1
  OR3/1 -> 1100/1
  AND/1 -> OR/1
  AND4/1 -> OR/2
  AND1/1 -> OR1/1
  AND5/1 -> OR1/2
  AND2/1 -> OR2/1
  AND6/1 -> OR2/2
  AND3/1 -> OR3/1
  AND7/1 -> OR3/2

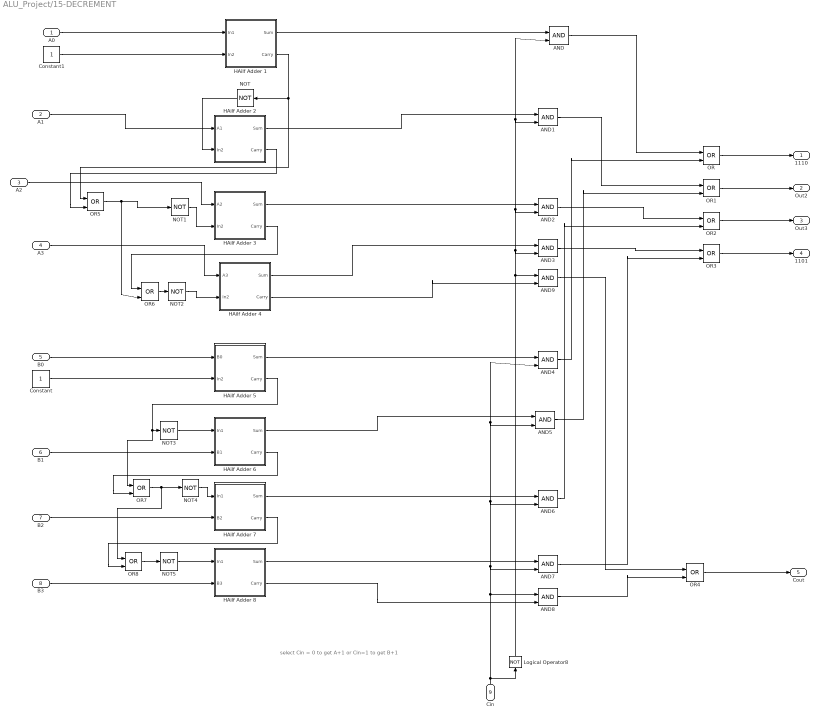
== system ALU_Project/15-DECREMENT ==
  note: select Cin = 0 to get A+1 or Cin=1 to get B+1
  A0 : Inport
  A1 : Inport  Port=2
  A2 : Inport  Port=3
  A3 : Inport  Port=4
  B0 : Inport  Port=5
  B1 : Inport  Port=6
  B2 : Inport  Port=7
  B3 : Inport  Port=8
  Cin : Inport  Port=9
  AND{,1..9} (10 alike) : Logic  IconShape=distinctive  AllPortsSameDT=off  OutDataTypeStr=boolean
  Constant : Constant
  Constant1 : Constant
  HAilf Adder 1 : Subsystem
  HAilf Adder 2 : Subsystem
  HAilf Adder 3 : Subsystem
  HAilf Adder 4 : Subsystem
  HAilf Adder 5 : Subsystem
  HAilf Adder 6 : Subsystem
  HAilf Adder 7 : Subsystem
  HAilf Adder 8 : Subsystem
  Logical Operator8 : Logic  Operator=NOT  IconShape=distinctive  AllPortsSameDT=off  OutDataTypeStr=boolean
  NOT{,1..5} (6 alike) : Logic  Operator=NOT  IconShape=distinctive  AllPortsSameDT=off  OutDataTypeStr=boolean
  OR{,1..8} (9 alike) : Logic  Operator=OR  IconShape=distinctive  AllPortsSameDT=off  OutDataTypeStr=boolean
  1110 : Outport
  Out2 : Outport  Port=2
  Out3 : Outport  Port=3
  1101 : Outport  Port=4
  Cout : Outport  Port=5
  wires:
  OR3/1 -> 1101/1
  AND2/1 -> OR2/1
  AND6/1 -> OR2/2
  OR2/1 -> Out3/1
  AND4/1 -> OR/2
  Cin/1 -> Logical Operator8/1, AND4/2, AND5/2, AND6/2, AND7/2, AND8/1
  AND5/1 -> OR1/2
  Logical Operator8/1 -> AND/2, AND1/2, AND2/2, AND3/2, AND9/1
  AND1/1 -> OR1/1
  OR1/1 -> Out2/1
  OR/1 -> 1110/1
  AND/1 -> OR/1
  AND3/1 -> OR3/1
  AND7/1 -> OR3/2
  HAilf Adder 2/1(Sum) -> AND1/1
  HAilf Adder 1/1(Sum) -> AND/1
  HAilf Adder 3/1(Sum) -> AND2/1
  HAilf Adder 4/1(Sum) -> AND3/1
  HAilf Adder 7/1(Sum) -> AND6/1
  HAilf Adder 8/1(Sum) -> AND7/1
  HAilf Adder 6/1(Sum) -> AND5/1
  HAilf Adder 5/1(Sum) -> AND4/1
  HAilf Adder 8/2(Carry) -> AND8/2
  A0/1 -> HAilf Adder 1/1(In1)
  A1/1 -> HAilf Adder 2/1(A1)
  A2/1 -> HAilf Adder 3/1(A2)
  A3/1 -> HAilf Adder 4/1(A3)
  B0/1 -> HAilf Adder 5/1(B0)
  B1/1 -> HAilf Adder 6/2(B1)
  B2/1 -> HAilf Adder 7/2(B2)
  B3/1 -> HAilf Adder 8/2(B3)
  Constant/1 -> HAilf Adder 5/2(In2)
  Constant1/1 -> HAilf Adder 1/2(In2)
  OR4/1 -> Cout/1
  HAilf Adder 4/2(Carry) -> AND9/2
  AND9/1 -> OR4/1
  AND8/1 -> OR4/2
  HAilf Adder 1/2(Carry) -> NOT/1, OR5/1
  NOT/1 -> HAilf Adder 2/2(In2)
  OR5/1 -> OR6/2, NOT1/1
  NOT1/1 -> HAilf Adder 3/2(In2)
  HAilf Adder 2/2(Carry) -> OR5/2
  NOT2/1 -> HAilf Adder 4/2(In2)
  OR6/1 -> NOT2/1
  HAilf Adder 3/2(Carry) -> OR6/1
  NOT3/1 -> HAilf Adder 6/1(In1)
  HAilf Adder 5/2(Carry) -> OR7/1, NOT3/1
  HAilf Adder 6/2(Carry) -> OR7/2
  OR7/1 -> OR8/1, NOT4/1
  NOT4/1 -> HAilf Adder 7/1(In1)
  NOT5/1 -> HAilf Adder 8/1(In1)
  HAilf Adder 7/2(Carry) -> OR8/2
  OR8/1 -> NOT5/1

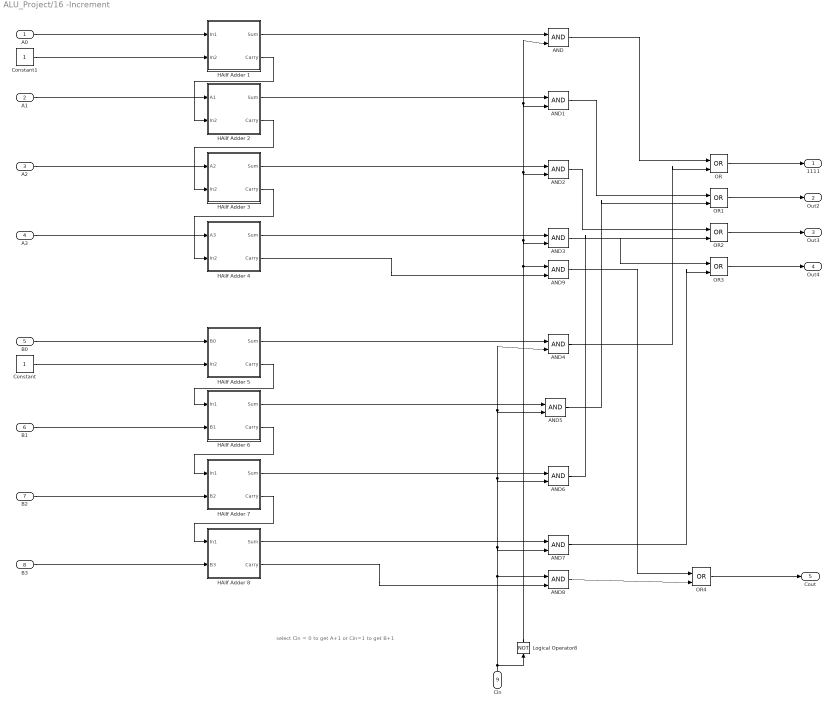
== system ALU_Project/16 -Increment ==
  note: select Cin = 0 to get A+1 or Cin=1 to get B+1
  A0 : Inport
  A1 : Inport  Port=2
  A2 : Inport  Port=3
  A3 : Inport  Port=4
  B0 : Inport  Port=5
  B1 : Inport  Port=6
  B2 : Inport  Port=7
  B3 : Inport  Port=8
  Cin : Inport  Port=9
  AND{,1..9} (10 alike) : Logic  IconShape=distinctive  AllPortsSameDT=off  OutDataTypeStr=boolean
  Constant : Constant
  Constant1 : Constant
  HAilf Adder 1 : Subsystem
  HAilf Adder 2 : Subsystem
  HAilf Adder 3 : Subsystem
  HAilf Adder 4 : Subsystem
  HAilf Adder 5 : Subsystem
  HAilf Adder 6 : Subsystem
  HAilf Adder 7 : Subsystem
  HAilf Adder 8 : Subsystem
  Logical Operator8 : Logic  Operator=NOT  IconShape=distinctive  AllPortsSameDT=off  OutDataTypeStr=boolean
  OR{,1..4} (5 alike) : Logic  Operator=OR  IconShape=distinctive  AllPortsSameDT=off  OutDataTypeStr=boolean
  1111 : Outport
  Out2 : Outport  Port=2
  Out3 : Outport  Port=3
  Out4 : Outport  Port=4
  Cout : Outport  Port=5
  wires:
  OR3/1 -> Out4/1
  AND2/1 -> OR2/1
  AND6/1 -> OR2/2
  OR2/1 -> Out3/1
  AND4/1 -> OR/2
  Cin/1 -> Logical Operator8/1, AND4/2, AND5/2, AND6/2, AND7/2, AND8/1
  AND5/1 -> OR1/2
  Logical Operator8/1 -> AND/2, AND1/2, AND2/2, AND3/2, AND9/1
  AND1/1 -> OR1/1
  OR1/1 -> Out2/1
  OR/1 -> 1111/1
  AND/1 -> OR/1
  AND3/1 -> OR3/1
  AND7/1 -> OR3/2
  HAilf Adder 2/1(Sum) -> AND1/1
  HAilf Adder 1/1(Sum) -> AND/1
  HAilf Adder 3/1(Sum) -> AND2/1
  HAilf Adder 4/1(Sum) -> AND3/1
  HAilf Adder 7/1(Sum) -> AND6/1
  HAilf Adder 8/1(Sum) -> AND7/1
  HAilf Adder 6/1(Sum) -> AND5/1
  HAilf Adder 5/1(Sum) -> AND4/1
  HAilf Adder 8/2(Carry) -> AND8/2
  HAilf Adder 5/2(Carry) -> HAilf Adder 6/1(In1)
  HAilf Adder 6/2(Carry) -> HAilf Adder 7/1(In1)
  HAilf Adder 7/2(Carry) -> HAilf Adder 8/1(In1)
  A0/1 -> HAilf Adder 1/1(In1)
  A1/1 -> HAilf Adder 2/1(A1)
  A2/1 -> HAilf Adder 3/1(A2)
  A3/1 -> HAilf Adder 4/1(A3)
  B0/1 -> HAilf Adder 5/1(B0)
  B1/1 -> HAilf Adder 6/2(B1)
  B2/1 -> HAilf Adder 7/2(B2)
  B3/1 -> HAilf Adder 8/2(B3)
  Constant/1 -> HAilf Adder 5/2(In2)
  Constant1/1 -> HAilf Adder 1/2(In2)
  HAilf Adder 1/2(Carry) -> HAilf Adder 2/2(In2)
  HAilf Adder 2/2(Carry) -> HAilf Adder 3/2(In2)
  HAilf Adder 3/2(Carry) -> HAilf Adder 4/2(In2)
  OR4/1 -> Cout/1
  HAilf Adder 4/2(Carry) -> AND9/2
  AND9/1 -> OR4/1
  AND8/1 -> OR4/2

== system ALU_Project/2 OR ==
  A0 : Inport
  A1 : Inport  Port=2
  A2 : Inport  Port=3
  A3 : Inport  Port=4
  B0 : Inport  Port=5
  B1 : Inport  Port=6
  B2 : Inport  Port=7
  B3 : Inport  Port=8
   {,1..3} (4 alike) : Logic  Operator=OR  AllPortsSameDT=off  OutDataTypeStr=boolean
  display{,1..3} (4 alike) : Display
  0001 : Outport
  Out2 : Outport  Port=2
  Out3 : Outport  Port=3
  Out4 : Outport  Port=4
  wires:
  B1/1 -> " 1"/2
  A2/1 -> " 2"/1
  B0/1 -> " "/2
  A3/1 -> " 3"/1
  B3/1 -> " 3"/2
  B2/1 -> " 2"/2
  A1/1 -> " 1"/1
  A0/1 -> " "/1
  " 1"/1 -> Out2/1, display1/1
  " 2"/1 -> Out3/1, display2/1
  " 3"/1 -> Out4/1, display3/1
  " "/1 -> 0001/1, display/1

== system ALU_Project/3 NOR ==
  A0 : Inport
  A1 : Inport  Port=2
  A2 : Inport  Port=3
  A3 : Inport  Port=4
  B0 : Inport  Port=5
  B1 : Inport  Port=6
  B2 : Inport  Port=7
  B3 : Inport  Port=8
   {,1..3} (4 alike) : Logic  Operator=NOR  AllPortsSameDT=off  OutDataTypeStr=boolean
  display{,1..3} (4 alike) : Display
  0010 : Outport
  Out2 : Outport  Port=2
  Out3 : Outport  Port=3
  Out4 : Outport  Port=4
  wires:
  A2/1 -> " 2"/1
  B3/1 -> " 3"/2
  B2/1 -> " 2"/2
  B1/1 -> " 1"/2
  B0/1 -> " "/2
  A3/1 -> " 3"/1
  A0/1 -> " "/1
  A1/1 -> " 1"/1
  " 3"/1 -> Out4/1, display3/1
  " 2"/1 -> Out3/1, display2/1
  " 1"/1 -> Out2/1, display1/1
  " "/1 -> 0010/1, display/1

== system ALU_Project/4 NAND ==
  A0 : Inport
  A1 : Inport  Port=2
  A2 : Inport  Port=3
  A3 : Inport  Port=4
  B0 : Inport  Port=5
  B1 : Inport  Port=6
  B2 : Inport  Port=7
  B3 : Inport  Port=8
   {,1..3} (4 alike) : Logic  Operator=NAND  AllPortsSameDT=off  OutDataTypeStr=boolean
  display{1..4} (4 alike) : Display
  0011 : Outport
  Out2 : Outport  Port=2
  Out3 : Outport  Port=3
  Out4 : Outport  Port=4
  wires:
  B1/1 -> " 2"/2
  A2/1 -> " 3"/1
  B0/1 -> " 1"/2
  A3/1 -> " "/1
  B3/1 -> " "/2
  B2/1 -> " 3"/2
  A1/1 -> " 2"/1
  A0/1 -> " 1"/1
  " 2"/1 -> Out2/1, display2/1
  " 3"/1 -> Out3/1, display3/1
  " "/1 -> Out4/1, display4/1
  " 1"/1 -> 0011/1, display1/1

== system ALU_Project/5 XOR ==
  A0 : Inport
  A1 : Inport  Port=2
  A2 : Inport  Port=3
  A3 : Inport  Port=4
  B0 : Inport  Port=5
  B1 : Inport  Port=6
  B2 : Inport  Port=7
  B3 : Inport  Port=8
   {,1..3} (4 alike) : Logic  Operator=XOR  AllPortsSameDT=off  OutDataTypeStr=boolean
  display{,1..3} (4 alike) : Display
  0100 : Outport
  Out2 : Outport  Port=2
  Out3 : Outport  Port=3
  0101 : Outport  Port=4
  wires:
  B1/1 -> " 1"/2
  A2/1 -> " 2"/1
  B0/1 -> " "/2
  A3/1 -> " 3"/1
  B3/1 -> " 3"/2
  B2/1 -> " 2"/2
  A1/1 -> " 1"/1
  A0/1 -> " "/1
  " 1"/1 -> Out2/1, display1/1
  " 2"/1 -> Out3/1, display2/1
  " 3"/1 -> 0101/1, display3/1
  " "/1 -> 0100/1, display/1

== system ALU_Project/6 XNOR ==
  A0 : Inport
  A1 : Inport  Port=2
  A2 : Inport  Port=3
  A3 : Inport  Port=4
  B0 : Inport  Port=5
  B1 : Inport  Port=6
  B2 : Inport  Port=7
  B3 : Inport  Port=8
   {,1..3} (4 alike) : Logic  Operator=NXOR  AllPortsSameDT=off  OutDataTypeStr=boolean
  display{,1..3} (4 alike) : Display
  0101 : Outport
  Out2 : Outport  Port=2
  Out3 : Outport  Port=3
  Out4 : Outport  Port=4
  wires:
  " 1"/1 -> Out2/1, display1/1
  " 2"/1 -> Out3/1, display2/1
  " 3"/1 -> Out4/1, display3/1
  " "/1 -> 0101/1, display/1
  B1/1 -> " 1"/2
  A2/1 -> " 2"/1
  B0/1 -> " "/2
  A3/1 -> " 3"/1
  B3/1 -> " 3"/2
  B2/1 -> " 2"/2
  A1/1 -> " 1"/1
  A0/1 -> " "/1

== system ALU_Project/7 - A SHFIT LEFT ==
  A0 : Inport
  A1 : Inport  Port=2
  A2 : Inport  Port=3
  A3 : Inport  Port=4
  CIN : Inport  Port=5
  Display{,1..9} (10 alike) : Display
  1 : Outport
  2 : Outport  Port=2
  3 : Outport  Port=3
  " 4" : Outport  Port=4
  COUT : Outport  Port=5
  wires:
  A3/1 -> Display9/1, Display4/1, COUT/1
  CIN/1 -> Display5/1, Display/1, 1/1
  A0/1 -> Display6/1, Display1/1, 2/1
  A1/1 -> Display7/1, Display2/1, 3/1
  A2/1 -> Display8/1, Display3/1, " 4"/1

== system ALU_Project/8 - SHIFT RIGHT A ==
  A0 : Inport
  A1 : Inport  Port=2
  A2 : Inport  Port=3
  A3 : Inport  Port=4
  CIN : Inport  Port=5
  0111 : Outport
  Out2 : Outport  Port=2
  Out3 : Outport  Port=3
  Out 4 : Outport  Port=4
  COUT : Outport  Port=5
  wires:
  A3/1 -> Out3/1
  CIN/1 -> Out 4/1
  A2/1 -> Out2/1
  A1/1 -> 0111/1
  A0/1 -> COUT/1

== system ALU_Project/9 - B SHIFT LEFT  ==
  B0 : Inport
  B1 : Inport  Port=2
  B2 : Inport  Port=3
  B3 : Inport  Port=4
  CIN : Inport  Port=5
  1000 : Outport
  Out2 : Outport  Port=2
  Out3 : Outport  Port=3
  Out 4 : Outport  Port=4
  COUT : Outport  Port=5
  wires:
  B3/1 -> COUT/1
  CIN/1 -> 1000/1
  B0/1 -> Out2/1
  B1/1 -> Out3/1
  B2/1 -> Out 4/1

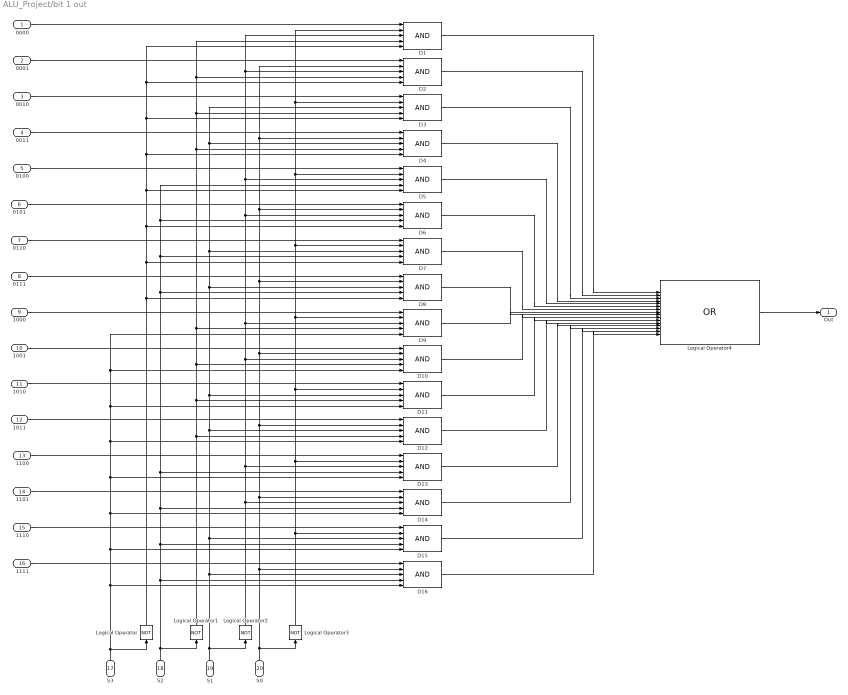
== system ALU_Project/bit 1 out ==
  0000 : Inport
  0001 : Inport  Port=2
  0010 : Inport  Port=3
  0011 : Inport  Port=4
  0100 : Inport  Port=5
  0101 : Inport  Port=6
  0110 : Inport  Port=7
  0111 : Inport  Port=8
  1000 : Inport  Port=9
  1001 : Inport  Port=10
  1010 : Inport  Port=11
  1011 : Inport  Port=12
  1100 : Inport  Port=13
  1101 : Inport  Port=14
  1110 : Inport  Port=15
  1111 : Inport  Port=16
  S3 : Inport  Port=17
  S2 : Inport  Port=18
  S1 : Inport  Port=19
  S0 : Inport  Port=20
  D{1..16} (16 alike) : Logic  Inputs=5  IconShape=distinctive  AllPortsSameDT=off  OutDataTypeStr=boolean
  Logical Operator{,1..3} (4 alike) : Logic  Operator=NOT  IconShape=distinctive  AllPortsSameDT=off  OutDataTypeStr=boolean
  Logical Operator4 : Logic  Operator=OR  Inputs=16  IconShape=distinctive  AllPortsSameDT=off  OutDataTypeStr=boolean
  Out : Outport
  wires:
  0000/1 -> D1/1
  0001/1 -> D2/1
  0010/1 -> D3/1
  0011/1 -> D4/1
  0100/1 -> D5/1
  0101/1 -> D6/1
  0110/1 -> D7/1
  0111/1 -> D8/1
  1000/1 -> D9/1
  1001/1 -> D10/1
  1010/1 -> D11/1
  1011/1 -> D12/1
  1100/1 -> D13/1
  1101/1 -> D14/1
  1110/1 -> D15/1
  1111/1 -> D16/1
  Logical Operator3/1 -> D15/2, D13/2, D11/2, D9/2, D7/2, D5/2, D3/2, D1/2
  S0/1 -> Logical Operator3/1, D16/2, D12/2, D10/2, D8/2, D2/2, D4/2, D6/2, D14/2
  Logical Operator2/1 -> D14/3, D13/3, D10/3, D9/3, D6/3, D5/3, D1/3, D2/3
  S1/1 -> Logical Operator2/1, D16/3, D15/3, D12/3, D11/3, D8/3, D7/3, D4/3, D3/3
  Logical Operator1/1 -> D4/4, D1/4, D2/4, D3/4, D9/4, D10/4, D11/4, D12/4
  S2/1 -> Logical Operator1/1, D16/4, D14/4, D7/4, D6/4, D5/4, D8/4, D13/4, D15/4
  Logical Operator/1 -> D7/5, D6/5, D4/5, D2/5, D1/5, D3/5, D5/5, D8/5
  S3/1 -> Logical Operator/1, D16/5, D10/5, D9/5, D11/5, D12/5, D13/5, D14/5, D15/5
  D1/1 -> Logical Operator4/1
  D2/1 -> Logical Operator4/2
  D3/1 -> Logical Operator4/3
  D4/1 -> Logical Operator4/4
  D5/1 -> Logical Operator4/5
  D6/1 -> Logical Operator4/6
  D7/1 -> Logical Operator4/7
  D8/1 -> Logical Operator4/8
  D9/1 -> Logical Operator4/9
  D11/1 -> Logical Operator4/11
  D10/1 -> Logical Operator4/10
  D12/1 -> Logical Operator4/12
  D13/1 -> Logical Operator4/13
  D14/1 -> Logical Operator4/14
  D15/1 -> Logical Operator4/15
  D16/1 -> Logical Operator4/16
  Logical Operator4/1 -> Out/1

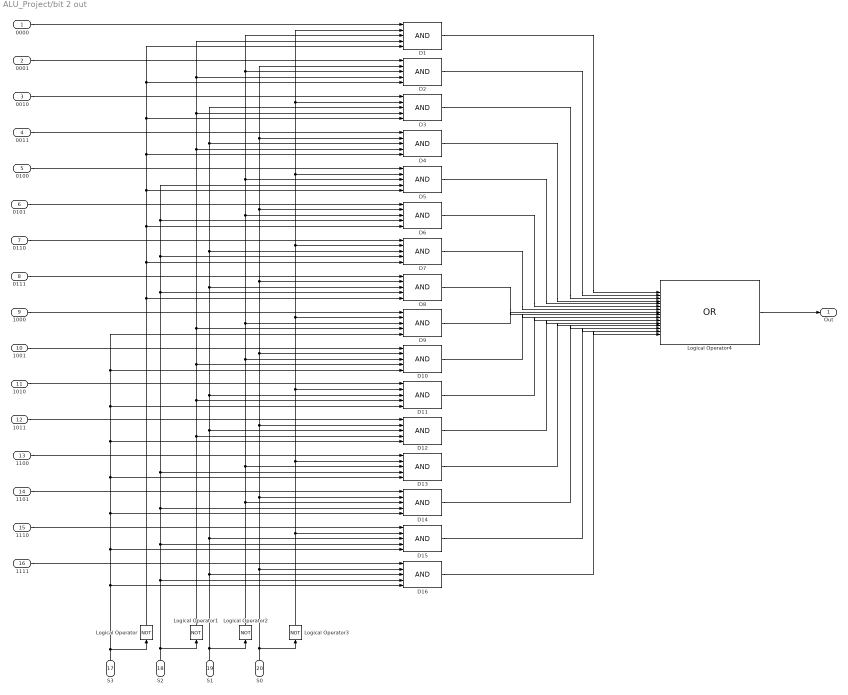
== system ALU_Project/bit 2 out ==
  0000 : Inport
  0001 : Inport  Port=2
  0010 : Inport  Port=3
  0011 : Inport  Port=4
  0100 : Inport  Port=5
  0101 : Inport  Port=6
  0110 : Inport  Port=7
  0111 : Inport  Port=8
  1000 : Inport  Port=9
  1001 : Inport  Port=10
  1010 : Inport  Port=11
  1011 : Inport  Port=12
  1100 : Inport  Port=13
  1101 : Inport  Port=14
  1110 : Inport  Port=15
  1111 : Inport  Port=16
  S3 : Inport  Port=17
  S2 : Inport  Port=18
  S1 : Inport  Port=19
  S0 : Inport  Port=20
  D{1..16} (16 alike) : Logic  Inputs=5  IconShape=distinctive  AllPortsSameDT=off  OutDataTypeStr=boolean
  Logical Operator{,1..3} (4 alike) : Logic  Operator=NOT  IconShape=distinctive  AllPortsSameDT=off  OutDataTypeStr=boolean
  Logical Operator4 : Logic  Operator=OR  Inputs=16  IconShape=distinctive  AllPortsSameDT=off  OutDataTypeStr=boolean
  Out : Outport
  wires:
  0000/1 -> D1/1
  0001/1 -> D2/1
  0010/1 -> D3/1
  0011/1 -> D4/1
  0100/1 -> D5/1
  0101/1 -> D6/1
  0110/1 -> D7/1
  0111/1 -> D8/1
  1000/1 -> D9/1
  1001/1 -> D10/1
  1010/1 -> D11/1
  1011/1 -> D12/1
  1100/1 -> D13/1
  1101/1 -> D14/1
  1110/1 -> D15/1
  1111/1 -> D16/1
  Logical Operator3/1 -> D15/2, D13/2, D11/2, D9/2, D7/2, D5/2, D3/2, D1/2
  S0/1 -> Logical Operator3/1, D16/2, D12/2, D10/2, D8/2, D2/2, D4/2, D6/2, D14/2
  Logical Operator2/1 -> D14/3, D13/3, D10/3, D9/3, D6/3, D5/3, D1/3, D2/3
  S1/1 -> Logical Operator2/1, D16/3, D15/3, D12/3, D11/3, D8/3, D7/3, D4/3, D3/3
  Logical Operator1/1 -> D4/4, D1/4, D2/4, D3/4, D9/4, D10/4, D11/4, D12/4
  S2/1 -> Logical Operator1/1, D16/4, D14/4, D7/4, D6/4, D5/4, D8/4, D13/4, D15/4
  Logical Operator/1 -> D7/5, D6/5, D4/5, D2/5, D1/5, D3/5, D5/5, D8/5
  S3/1 -> Logical Operator/1, D16/5, D10/5, D9/5, D11/5, D12/5, D13/5, D14/5, D15/5
  D1/1 -> Logical Operator4/1
  D2/1 -> Logical Operator4/2
  D3/1 -> Logical Operator4/3
  D4/1 -> Logical Operator4/4
  D5/1 -> Logical Operator4/5
  D6/1 -> Logical Operator4/6
  D7/1 -> Logical Operator4/7
  D8/1 -> Logical Operator4/8
  D9/1 -> Logical Operator4/9
  D11/1 -> Logical Operator4/11
  D10/1 -> Logical Operator4/10
  D12/1 -> Logical Operator4/12
  D13/1 -> Logical Operator4/13
  D14/1 -> Logical Operator4/14
  D15/1 -> Logical Operator4/15
  D16/1 -> Logical Operator4/16
  Logical Operator4/1 -> Out/1

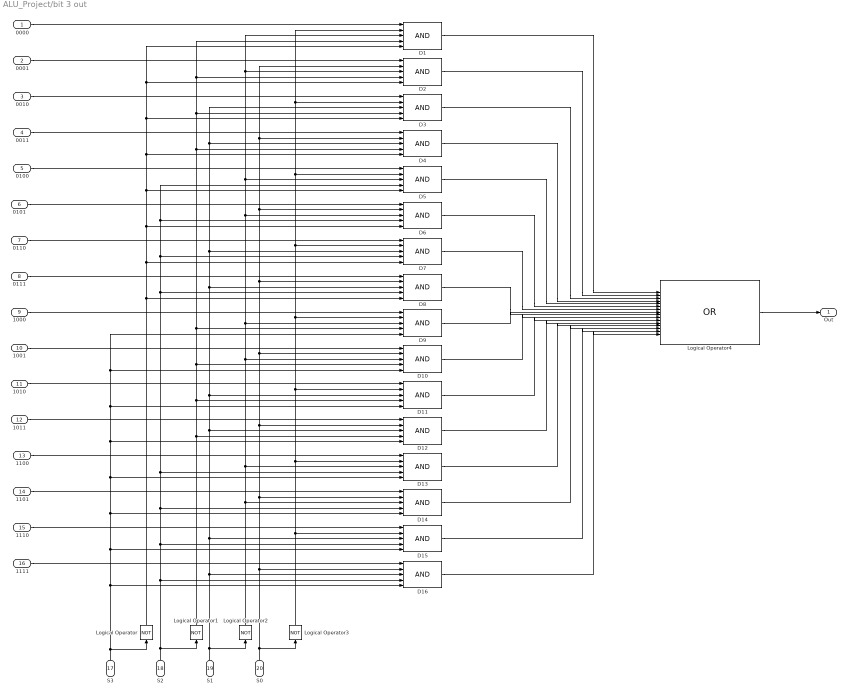
== system ALU_Project/bit 3 out ==
  0000 : Inport
  0001 : Inport  Port=2
  0010 : Inport  Port=3
  0011 : Inport  Port=4
  0100 : Inport  Port=5
  0101 : Inport  Port=6
  0110 : Inport  Port=7
  0111 : Inport  Port=8
  1000 : Inport  Port=9
  1001 : Inport  Port=10
  1010 : Inport  Port=11
  1011 : Inport  Port=12
  1100 : Inport  Port=13
  1101 : Inport  Port=14
  1110 : Inport  Port=15
  1111 : Inport  Port=16
  S3 : Inport  Port=17
  S2 : Inport  Port=18
  S1 : Inport  Port=19
  S0 : Inport  Port=20
  D{1..16} (16 alike) : Logic  Inputs=5  IconShape=distinctive  AllPortsSameDT=off  OutDataTypeStr=boolean
  Logical Operator{,1..3} (4 alike) : Logic  Operator=NOT  IconShape=distinctive  AllPortsSameDT=off  OutDataTypeStr=boolean
  Logical Operator4 : Logic  Operator=OR  Inputs=16  IconShape=distinctive  AllPortsSameDT=off  OutDataTypeStr=boolean
  Out : Outport
  wires:
  0000/1 -> D1/1
  0001/1 -> D2/1
  0010/1 -> D3/1
  0011/1 -> D4/1
  0100/1 -> D5/1
  0101/1 -> D6/1
  0110/1 -> D7/1
  0111/1 -> D8/1
  1000/1 -> D9/1
  1001/1 -> D10/1
  1010/1 -> D11/1
  1011/1 -> D12/1
  1100/1 -> D13/1
  1101/1 -> D14/1
  1110/1 -> D15/1
  1111/1 -> D16/1
  Logical Operator3/1 -> D15/2, D13/2, D11/2, D9/2, D7/2, D5/2, D3/2, D1/2
  S0/1 -> Logical Operator3/1, D16/2, D12/2, D10/2, D8/2, D2/2, D4/2, D6/2, D14/2
  Logical Operator2/1 -> D14/3, D13/3, D10/3, D9/3, D6/3, D5/3, D1/3, D2/3
  S1/1 -> Logical Operator2/1, D16/3, D15/3, D12/3, D11/3, D8/3, D7/3, D4/3, D3/3
  Logical Operator1/1 -> D4/4, D1/4, D2/4, D3/4, D9/4, D10/4, D11/4, D12/4
  S2/1 -> Logical Operator1/1, D16/4, D14/4, D7/4, D6/4, D5/4, D8/4, D13/4, D15/4
  Logical Operator/1 -> D7/5, D6/5, D4/5, D2/5, D1/5, D3/5, D5/5, D8/5
  S3/1 -> Logical Operator/1, D16/5, D10/5, D9/5, D11/5, D12/5, D13/5, D14/5, D15/5
  D1/1 -> Logical Operator4/1
  D2/1 -> Logical Operator4/2
  D3/1 -> Logical Operator4/3
  D4/1 -> Logical Operator4/4
  D5/1 -> Logical Operator4/5
  D6/1 -> Logical Operator4/6
  D7/1 -> Logical Operator4/7
  D8/1 -> Logical Operator4/8
  D9/1 -> Logical Operator4/9
  D11/1 -> Logical Operator4/11
  D10/1 -> Logical Operator4/10
  D12/1 -> Logical Operator4/12
  D13/1 -> Logical Operator4/13
  D14/1 -> Logical Operator4/14
  D15/1 -> Logical Operator4/15
  D16/1 -> Logical Operator4/16
  Logical Operator4/1 -> Out/1

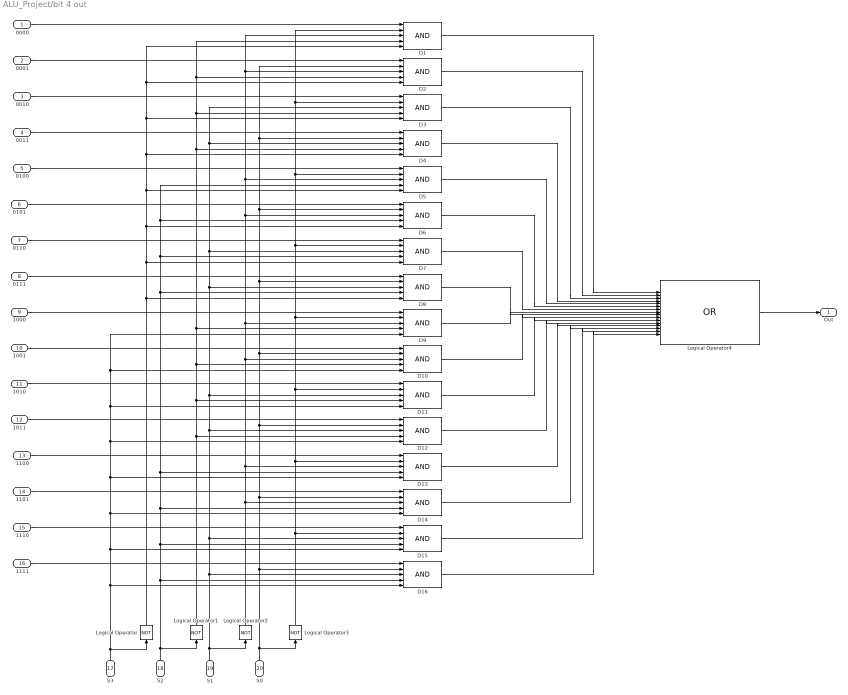
== system ALU_Project/bit 4 out ==
  0000 : Inport
  0001 : Inport  Port=2
  0010 : Inport  Port=3
  0011 : Inport  Port=4
  0100 : Inport  Port=5
  0101 : Inport  Port=6
  0110 : Inport  Port=7
  0111 : Inport  Port=8
  1000 : Inport  Port=9
  1001 : Inport  Port=10
  1010 : Inport  Port=11
  1011 : Inport  Port=12
  1100 : Inport  Port=13
  1101 : Inport  Port=14
  1110 : Inport  Port=15
  1111 : Inport  Port=16
  S3 : Inport  Port=17
  S2 : Inport  Port=18
  S1 : Inport  Port=19
  S0 : Inport  Port=20
  D{1..16} (16 alike) : Logic  Inputs=5  IconShape=distinctive  AllPortsSameDT=off  OutDataTypeStr=boolean
  Logical Operator{,1..3} (4 alike) : Logic  Operator=NOT  IconShape=distinctive  AllPortsSameDT=off  OutDataTypeStr=boolean
  Logical Operator4 : Logic  Operator=OR  Inputs=16  IconShape=distinctive  AllPortsSameDT=off  OutDataTypeStr=boolean
  Out : Outport
  wires:
  0000/1 -> D1/1
  0001/1 -> D2/1
  0010/1 -> D3/1
  0011/1 -> D4/1
  0100/1 -> D5/1
  0101/1 -> D6/1
  0110/1 -> D7/1
  0111/1 -> D8/1
  1000/1 -> D9/1
  1001/1 -> D10/1
  1010/1 -> D11/1
  1011/1 -> D12/1
  1100/1 -> D13/1
  1101/1 -> D14/1
  1110/1 -> D15/1
  1111/1 -> D16/1
  Logical Operator3/1 -> D15/2, D13/2, D11/2, D9/2, D7/2, D5/2, D3/2, D1/2
  S0/1 -> Logical Operator3/1, D16/2, D12/2, D10/2, D8/2, D2/2, D4/2, D6/2, D14/2
  Logical Operator2/1 -> D14/3, D13/3, D10/3, D9/3, D6/3, D5/3, D1/3, D2/3
  S1/1 -> Logical Operator2/1, D16/3, D15/3, D12/3, D11/3, D8/3, D7/3, D4/3, D3/3
  Logical Operator1/1 -> D4/4, D1/4, D2/4, D3/4, D9/4, D10/4, D11/4, D12/4
  S2/1 -> Logical Operator1/1, D16/4, D14/4, D7/4, D6/4, D5/4, D8/4, D13/4, D15/4
  Logical Operator/1 -> D7/5, D6/5, D4/5, D2/5, D1/5, D3/5, D5/5, D8/5
  S3/1 -> Logical Operator/1, D16/5, D10/5, D9/5, D11/5, D12/5, D13/5, D14/5, D15/5
  D1/1 -> Logical Operator4/1
  D2/1 -> Logical Operator4/2
  D3/1 -> Logical Operator4/3
  D4/1 -> Logical Operator4/4
  D5/1 -> Logical Operator4/5
  D6/1 -> Logical Operator4/6
  D7/1 -> Logical Operator4/7
  D8/1 -> Logical Operator4/8
  D9/1 -> Logical Operator4/9
  D11/1 -> Logical Operator4/11
  D10/1 -> Logical Operator4/10
  D12/1 -> Logical Operator4/12
  D13/1 -> Logical Operator4/13
  D14/1 -> Logical Operator4/14
  D15/1 -> Logical Operator4/15
  D16/1 -> Logical Operator4/16
  Logical Operator4/1 -> Out/1

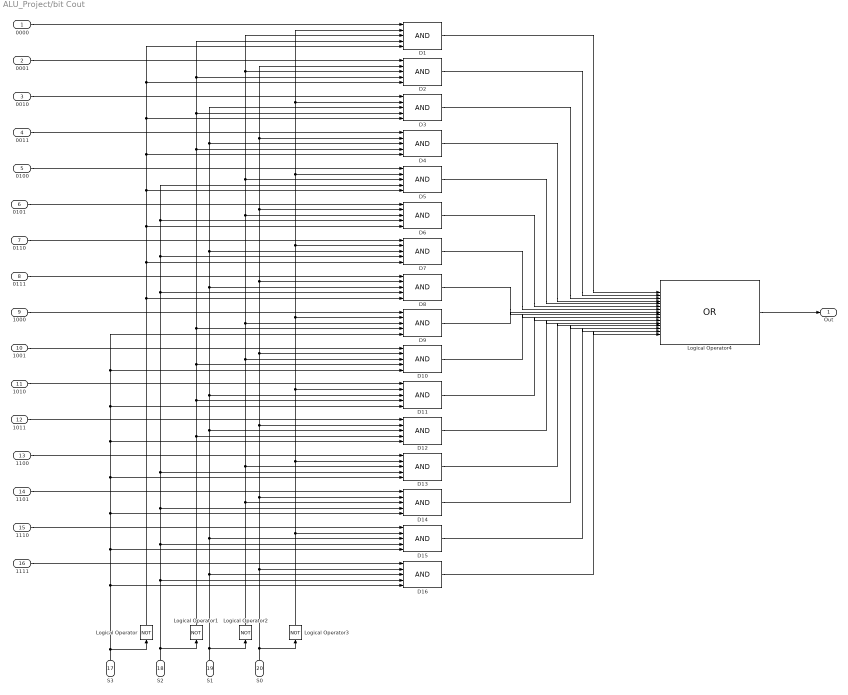
== system ALU_Project/bit Cout ==
  0000 : Inport
  0001 : Inport  Port=2
  0010 : Inport  Port=3
  0011 : Inport  Port=4
  0100 : Inport  Port=5
  0101 : Inport  Port=6
  0110 : Inport  Port=7
  0111 : Inport  Port=8
  1000 : Inport  Port=9
  1001 : Inport  Port=10
  1010 : Inport  Port=11
  1011 : Inport  Port=12
  1100 : Inport  Port=13
  1101 : Inport  Port=14
  1110 : Inport  Port=15
  1111 : Inport  Port=16
  S3 : Inport  Port=17
  S2 : Inport  Port=18
  S1 : Inport  Port=19
  S0 : Inport  Port=20
  D{1..16} (16 alike) : Logic  Inputs=5  IconShape=distinctive  AllPortsSameDT=off  OutDataTypeStr=boolean
  Logical Operator{,1..3} (4 alike) : Logic  Operator=NOT  IconShape=distinctive  AllPortsSameDT=off  OutDataTypeStr=boolean
  Logical Operator4 : Logic  Operator=OR  Inputs=16  IconShape=distinctive  AllPortsSameDT=off  OutDataTypeStr=boolean
  Out : Outport
  wires:
  0000/1 -> D1/1
  0001/1 -> D2/1
  0010/1 -> D3/1
  0011/1 -> D4/1
  0100/1 -> D5/1
  0101/1 -> D6/1
  0110/1 -> D7/1
  0111/1 -> D8/1
  1000/1 -> D9/1
  1001/1 -> D10/1
  1010/1 -> D11/1
  1011/1 -> D12/1
  1100/1 -> D13/1
  1101/1 -> D14/1
  1110/1 -> D15/1
  1111/1 -> D16/1
  Logical Operator3/1 -> D15/2, D13/2, D11/2, D9/2, D7/2, D5/2, D3/2, D1/2
  S0/1 -> Logical Operator3/1, D16/2, D12/2, D10/2, D8/2, D2/2, D4/2, D6/2, D14/2
  Logical Operator2/1 -> D14/3, D13/3, D10/3, D9/3, D6/3, D5/3, D1/3, D2/3
  S1/1 -> Logical Operator2/1, D16/3, D15/3, D12/3, D11/3, D8/3, D7/3, D4/3, D3/3
  Logical Operator1/1 -> D4/4, D1/4, D2/4, D3/4, D9/4, D10/4, D11/4, D12/4
  S2/1 -> Logical Operator1/1, D16/4, D14/4, D7/4, D6/4, D5/4, D8/4, D13/4, D15/4
  Logical Operator/1 -> D7/5, D6/5, D4/5, D2/5, D1/5, D3/5, D5/5, D8/5
  S3/1 -> Logical Operator/1, D16/5, D10/5, D9/5, D11/5, D12/5, D13/5, D14/5, D15/5
  D1/1 -> Logical Operator4/1
  D2/1 -> Logical Operator4/2
  D3/1 -> Logical Operator4/3
  D4/1 -> Logical Operator4/4
  D5/1 -> Logical Operator4/5
  D6/1 -> Logical Operator4/6
  D7/1 -> Logical Operator4/7
  D8/1 -> Logical Operator4/8
  D9/1 -> Logical Operator4/9
  D11/1 -> Logical Operator4/11
  D10/1 -> Logical Operator4/10
  D12/1 -> Logical Operator4/12
  D13/1 -> Logical Operator4/13
  D14/1 -> Logical Operator4/14
  D15/1 -> Logical Operator4/15
  D16/1 -> Logical Operator4/16
  Logical Operator4/1 -> Out/1
